simulink model "LineToGotoFrom_Cover"  (R2016b)
settings: Solver=VariableStepAuto  StartTime=0.0  StopTime=10.0  RelTol=1e-3
settings Model: Creator=monika  LastModifiedBy=monika

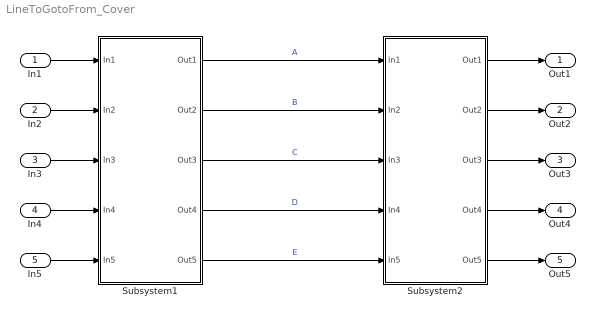
== system LineToGotoFrom_Cover ==
  In1 : Inport
  In2 : Inport  Port=2
  In3 : Inport  Port=3
  In4 : Inport  Port=4
  In5 : Inport  Port=5
  Subsystem1 : Subsystem
  Subsystem2 : Subsystem
  Out1 : Outport
  Out2 : Outport  Port=2
  Out3 : Outport  Port=3
  Out4 : Outport  Port=4
  Out5 : Outport  Port=5
  wires:
  Subsystem2/1(Out1) -> Out1/1
  Subsystem2/2(Out2) -> Out2/1
  Subsystem2/3(Out3) -> Out3/1
  Subsystem2/4(Out4) -> Out4/1
  Subsystem2/5(Out5) -> Out5/1
  In1/1 -> Subsystem1/1(In1)
  In2/1 -> Subsystem1/2(In2)
  In3/1 -> Subsystem1/3(In3)
  In4/1 -> Subsystem1/4(In4)
  In5/1 -> Subsystem1/5(In5)
  Subsystem1/1(Out1) -> Subsystem2/1(In1)  "A"
  Subsystem1/2(Out2) -> Subsystem2/2(In2)  "B"
  Subsystem1/3(Out3) -> Subsystem2/3(In3)  "C"
  Subsystem1/4(Out4) -> Subsystem2/4(In4)  "D"
  Subsystem1/5(Out5) -> Subsystem2/5(In5)  "E"

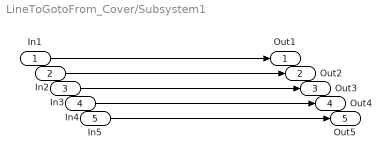
== system LineToGotoFrom_Cover/Subsystem1 ==
  In1 : Inport
  In2 : Inport  Port=2
  In3 : Inport  Port=3
  In4 : Inport  Port=4
  In5 : Inport  Port=5
  Out1 : Outport
  Out2 : Outport  Port=2
  Out3 : Outport  Port=3
  Out4 : Outport  Port=4
  Out5 : Outport  Port=5
  wires:
  In1/1 -> Out1/1
  In2/1 -> Out2/1
  In3/1 -> Out3/1
  In4/1 -> Out4/1
  In5/1 -> Out5/1

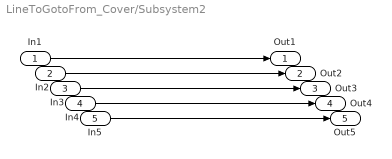
== system LineToGotoFrom_Cover/Subsystem2 ==
  In1 : Inport
  In2 : Inport  Port=2
  In3 : Inport  Port=3
  In4 : Inport  Port=4
  In5 : Inport  Port=5
  Out1 : Outport
  Out2 : Outport  Port=2
  Out3 : Outport  Port=3
  Out4 : Outport  Port=4
  Out5 : Outport  Port=5
  wires:
  In1/1 -> Out1/1
  In2/1 -> Out2/1
  In3/1 -> Out3/1
  In4/1 -> Out4/1
  In5/1 -> Out5/1
